simulink model "TODE"  (Simulink 8.7)
settings: Solver=VariableStepAuto  StartTime=0.0  StopTime=10.0  RelTol=1e-3
settings Model: Creator=Administrator  LastModifiedBy=Administrator
settings DataIOCC: LimitDataPoints=off  SaveFormat=Dataset
settings DebuggingCC: UnderspecifiedInitializationDetection=Simplified  MergeDetectMultiDrivingBlocksExec=error
settings HardwareCC: ProdBitPerChar=16  ProdBitPerInt=16  ProdLargestAtomicInteger=Integer  ProdIntDivRoundTo=Zero  ProdEndianess=LittleEndian  ProdWordSize=16  ProdHWDeviceType=Texas Instruments->C2000
settings ModelReferenceCC: PropagateSignalLabelsOutOfModel=on
settings ConfigComp: CovModelRefEnable=off

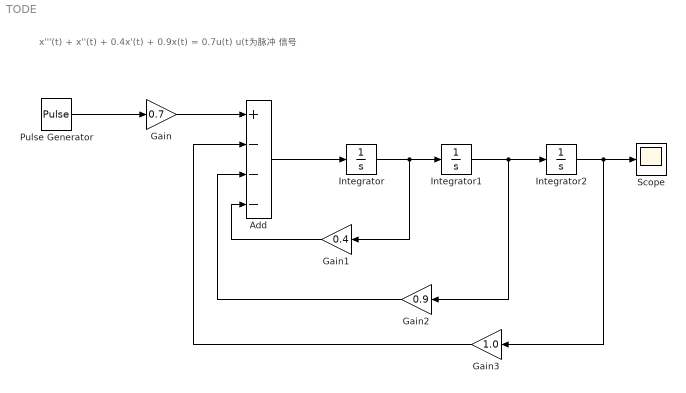
== system TODE ==
  note: x'''(t) + x''(t) + 0.4x'(t) + 0.9x(t) = 0.7u(t)
      | u(t)为脉冲 信号
  Add : Sum  Inputs=+---
  Gain : Gain  Gain=0.7
  Gain1 : Gain  Gain=0.4
  Gain2 : Gain  Gain=0.9
  Gain3 : Gain  Gain=1.0
  Integrator : Integrator  InitialCondition=0.01
  Integrator1 : Integrator  InitialCondition=0.01
  Integrator2 : Integrator  InitialCondition=0.01
  Pulse Generator : DiscretePulseGenerator  PulseType=Time based  PulseWidth=5
  Scope : Scope
  wires:
  Pulse Generator/1 -> Gain/1
  Gain/1 -> Add/1
  Integrator/1 -> Gain1/1, Integrator1/1
  Integrator1/1 -> Gain2/1, Integrator2/1
  Add/1 -> Integrator/1
  Integrator2/1 -> Gain3/1, Scope/1
  Gain1/1 -> Add/4
  Gain2/1 -> Add/3
  Gain3/1 -> Add/2
